simulink model "positionWalking_legacy"  (Simulink 8.3)
settings: Solver=FixedStepDiscrete  StartTime=0.0  StopTime=Config.t_end  FixedStep=Config.t_step  RelTol=1e-3
InitFcn:
  | cd(fileparts(which(bdroot)));
  | initTorqueWalking;
undefined symbols (not defined in the file): Config, DiscIntNeverNeededParam, gains, ROBOT_DOF
libraries: WBToolboxLibrary x88
(part 1 of 3)
settings Model: Creator=gnava  LastModifiedBy=gabri
settings DataIOCC: LimitDataPoints=off  SaveFormat=StructureWithTime  SignalLoggingSaveFormat=Dataset
settings DebuggingCC: UnderspecifiedInitializationDetection=Simplified  MergeDetectMultiDrivingBlocksExec=error  SolverPrmCheckMsg=none  FrameProcessingCompatibilityMsg=error  StateNameClashWarn=none  SFUnexpectedBacktrackingDiag=error  SFNoUnconditionalDefaultTransitionDiag=error
settings HardwareCC: ProdBitPerPointer=64  ProdLargestAtomicFloat=Float  ProdIntDivRoundTo=Zero  ProdEndianess=LittleEndian  ProdHWDeviceType=Specified
settings ModelReferenceCC: PropagateSignalLabelsOutOfModel=on
settings GRTTargetCC: TargetLangStandard=C99 (ISO)  GeneratePreprocessorConditionals=Use local settings  CombineOutputUpdateFcns=on  GRTInterface=off

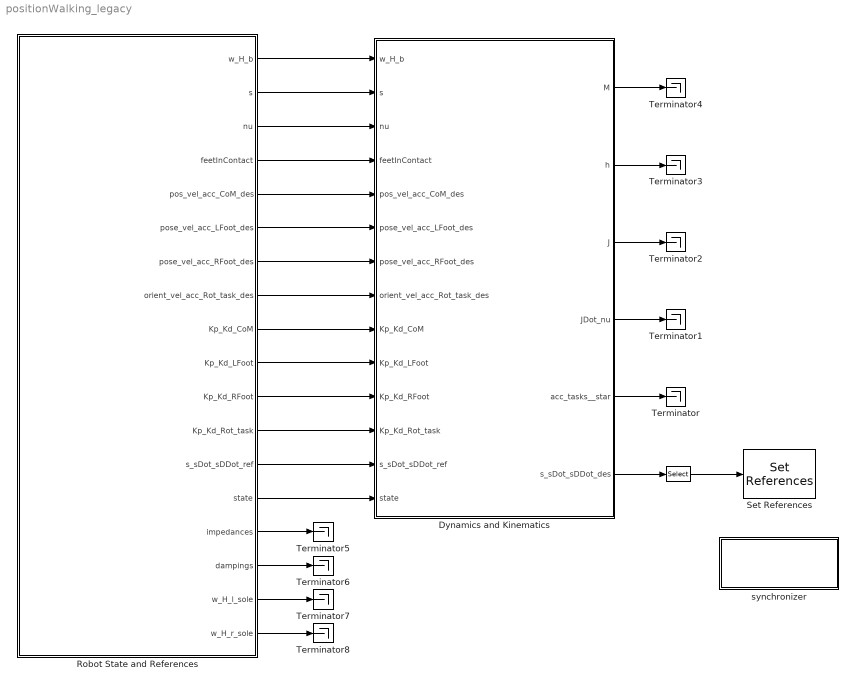
== system positionWalking_legacy ==
  "  " : Selector  NumberOfDimensions=2  InputPortWidth=ROBOT_DOF+16  IndexOptions=Index vector (dialog),Index vector (dialog)  Indices=[1:ROBOT_DOF],[1]  OutputSizes=1,1
  Dynamics and Kinematics : Subsystem
  Robot State and References : Subsystem
  Set References : WBToolboxLibrary/wholeBodyActuators/Set References  controlType=Position Direct  fullOrSubControl=Full  controlledJoints=''  robotName=WBT_robotName  localName=WBT_modelName  wbiFile=WBT_wbiFilename  wbiList=WBT_wbiList
  Terminator{,1..8} (9 alike) : Terminator
  synchronizer : Subsystem
      mask Display: disp('SYNCHRONIZER')
  wires:
  "  "/1 -> Set References/1
  Robot State and References/1(w_H_b) -> Dynamics and Kinematics/1(w_H_b)
  Robot State and References/2(s) -> Dynamics and Kinematics/2(s)
  Robot State and References/3(nu) -> Dynamics and Kinematics/3(nu)
  Robot State and References/4(feetInContact) -> Dynamics and Kinematics/4(feetInContact)
  Robot State and References/5(pos_vel_acc_CoM_des) -> Dynamics and Kinematics/5(pos_vel_acc_CoM_des)
  Robot State and References/6(pose_vel_acc_LFoot_des) -> Dynamics and Kinematics/6(pose_vel_acc_LFoot_des)
  Robot State and References/7(pose_vel_acc_RFoot_des) -> Dynamics and Kinematics/7(pose_vel_acc_RFoot_des)
  Robot State and References/8(orient_vel_acc_Rot_task_des) -> Dynamics and Kinematics/8(orient_vel_acc_Rot_task_des)
  Robot State and References/9(Kp_Kd_CoM) -> Dynamics and Kinematics/9(Kp_Kd_CoM)
  Robot State and References/10(Kp_Kd_LFoot) -> Dynamics and Kinematics/10(Kp_Kd_LFoot)
  Robot State and References/11(Kp_Kd_RFoot) -> Dynamics and Kinematics/11(Kp_Kd_RFoot)
  Robot State and References/12(Kp_Kd_Rot_task) -> Dynamics and Kinematics/12(Kp_Kd_Rot_task)
  Robot State and References/13(s_sDot_sDDot_ref) -> Dynamics and Kinematics/13(s_sDot_sDDot_ref)
  Robot State and References/14(state) -> Dynamics and Kinematics/14(state)
  Robot State and References/15(impedances) -> Terminator5/1
  Robot State and References/16(dampings) -> Terminator6/1
  Robot State and References/17(w_H_l_sole) -> Terminator7/1
  Robot State and References/18(w_H_r_sole) -> Terminator8/1
  Dynamics and Kinematics/6(s_sDot_sDDot_des) -> "  "/1
  Dynamics and Kinematics/5(acc_tasks__star) -> Terminator/1
  Dynamics and Kinematics/4(JDot_nu) -> Terminator1/1
  Dynamics and Kinematics/3(J) -> Terminator2/1
  Dynamics and Kinematics/2(h) -> Terminator3/1
  Dynamics and Kinematics/1(M) -> Terminator4/1

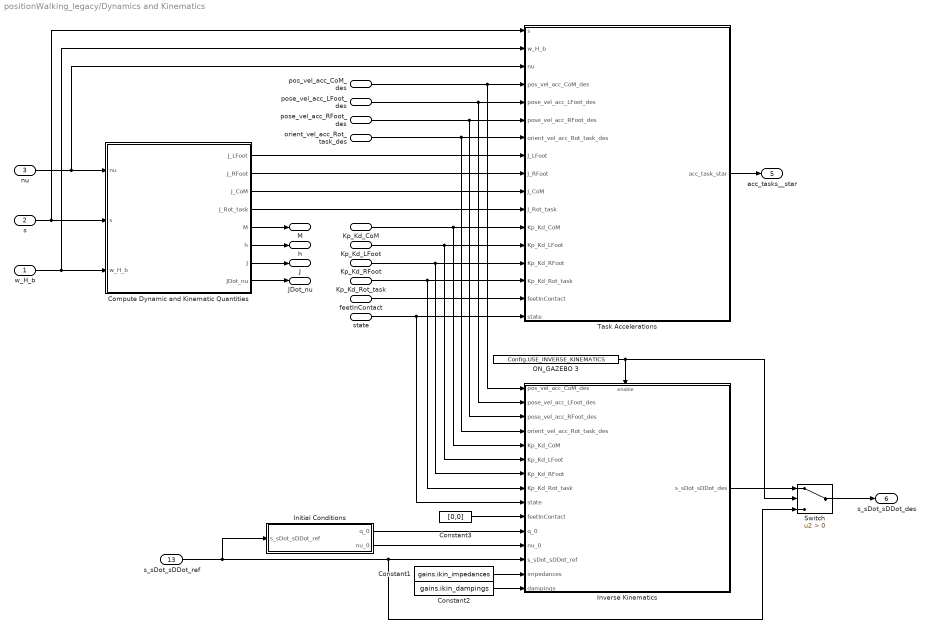
== system positionWalking_legacy/Dynamics and Kinematics ==
  w_H_b : Inport
  s : Inport  Port=2
  nu : Inport  Port=3
  feetInContact : Inport  Port=4
  pos_vel_acc_CoM_des : Inport  Port=5
  pose_vel_acc_LFoot_des : Inport  Port=6
  pose_vel_acc_RFoot_des : Inport  Port=7
  orient_vel_acc_Rot_task_des : Inport  Port=8
  Kp_Kd_CoM : Inport  Port=9
  Kp_Kd_LFoot : Inport  Port=10
  Kp_Kd_RFoot : Inport  Port=11
  Kp_Kd_Rot_task : Inport  Port=12
  s_sDot_sDDot_ref : Inport  Port=13
  state : Inport  Port=14
  Compute Dynamic and Kinematic Quantities : Subsystem
  Constant1 : Constant  Value=gains.ikin_impedances
  Constant2 : Constant  Value=gains.ikin_dampings
  Constant3 : Constant  Value=[0,0]
  Initial Conditions : Subsystem
  Inverse Kinematics : Subsystem
  ON_GAZEBO 3 : Constant  Value=Config.USE_INVERSE_KINEMATICS
  Switch : Switch  Criteria=u2 > Threshold
  Task Accelerations : Subsystem
  M : Outport
  h : Outport  Port=2
  J : Outport  Port=3
  JDot_nu : Outport  Port=4
  acc_tasks__star : Outport  Port=5
  s_sDot_sDDot_des : Outport  Port=6
  wires:
  pos_vel_acc_CoM_des/1 -> Inverse Kinematics/1(pos_vel_acc_CoM_des), Task Accelerations/4(pos_vel_acc_CoM_des)
  pose_vel_acc_LFoot_des/1 -> Inverse Kinematics/2(pose_vel_acc_LFoot_des), Task Accelerations/5(pose_vel_acc_LFoot_des)
  pose_vel_acc_RFoot_des/1 -> Inverse Kinematics/3(pose_vel_acc_RFoot_des), Task Accelerations/6(pose_vel_acc_RFoot_des)
  orient_vel_acc_Rot_task_des/1 -> Inverse Kinematics/4(orient_vel_acc_Rot_task_des), Task Accelerations/7(orient_vel_acc_Rot_task_des)
  Kp_Kd_CoM/1 -> Inverse Kinematics/5(Kp_Kd_CoM), Task Accelerations/12(Kp_Kd_CoM)
  Kp_Kd_LFoot/1 -> Inverse Kinematics/6(Kp_Kd_LFoot), Task Accelerations/13(Kp_Kd_LFoot)
  Kp_Kd_RFoot/1 -> Inverse Kinematics/7(Kp_Kd_RFoot), Task Accelerations/14(Kp_Kd_RFoot)
  Kp_Kd_Rot_task/1 -> Inverse Kinematics/8(Kp_Kd_Rot_task), Task Accelerations/15(Kp_Kd_Rot_task)
  feetInContact/1 -> Task Accelerations/16(feetInContact)
  Task Accelerations/1(acc_task_star) -> acc_tasks__star/1
  ON_GAZEBO 3/1 -> Switch/2, Inverse Kinematics/Enable
  Inverse Kinematics/1(s_sDot_sDDot_des) -> Switch/1
  state/1 -> Inverse Kinematics/9(state), Task Accelerations/17(state)
  nu/1 -> Compute Dynamic and Kinematic Quantities/1(nu), Task Accelerations/3(nu)
  s/1 -> Task Accelerations/1(s), Compute Dynamic and Kinematic Quantities/2(s)
  w_H_b/1 -> Compute Dynamic and Kinematic Quantities/3(w_H_b), Task Accelerations/2(w_H_b)
  Compute Dynamic and Kinematic Quantities/6(h) -> h/1
  Compute Dynamic and Kinematic Quantities/1(J_LFoot) -> Task Accelerations/8(J_LFoot)
  Compute Dynamic and Kinematic Quantities/2(J_RFoot) -> Task Accelerations/9(J_RFoot)
  Compute Dynamic and Kinematic Quantities/3(J_CoM) -> Task Accelerations/10(J_CoM)
  Compute Dynamic and Kinematic Quantities/5(M) -> M/1
  Compute Dynamic and Kinematic Quantities/4(J_Rot_task) -> Task Accelerations/11(J_Rot_task)
  Compute Dynamic and Kinematic Quantities/7(J) -> J/1
  Compute Dynamic and Kinematic Quantities/8(JDot_nu) -> JDot_nu/1
  s_sDot_sDDot_ref/1 -> Inverse Kinematics/13(s_sDot_sDDot_ref), Switch/3, Initial Conditions/1(s_sDot_sDDot_ref)
  Initial Conditions/1(q_0) -> Inverse Kinematics/11(q_0)
  Initial Conditions/2(nu_0) -> Inverse Kinematics/12(nu_0)
  Constant1/1 -> Inverse Kinematics/14(impedances)
  Constant2/1 -> Inverse Kinematics/15(dampings)
  Switch/1 -> s_sDot_sDDot_des/1
  Constant3/1 -> Inverse Kinematics/10(feetInContact)

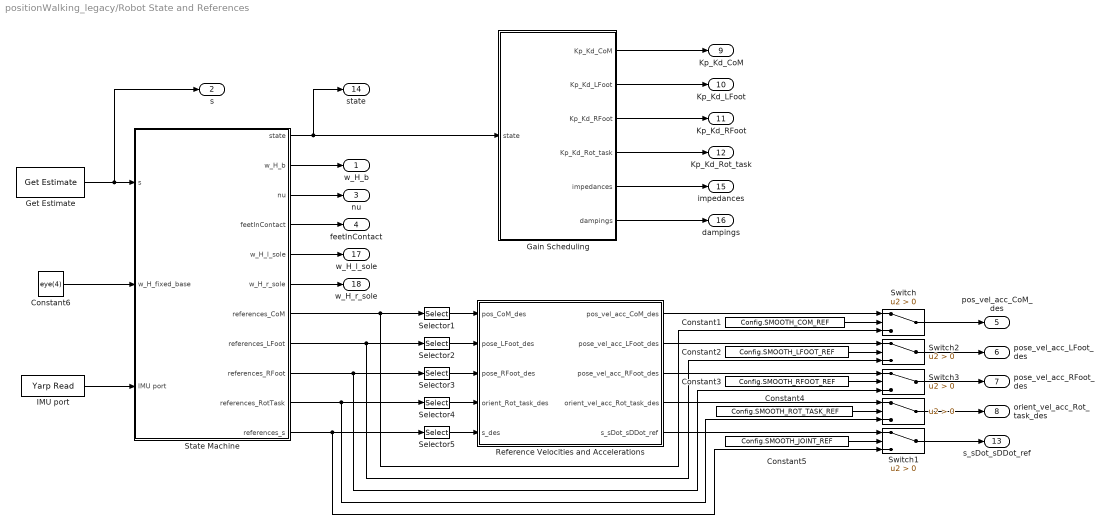
== system positionWalking_legacy/Robot State and References ==
  " " : Switch  Criteria=u2 > Threshold
  Constant1 : Constant  Value=Config.SMOOTH_COM_REF
  Constant2 : Constant  Value=Config.SMOOTH_LFOOT_REF
  Constant3 : Constant  Value=Config.SMOOTH_RFOOT_REF
  Constant4 : Constant  Value=Config.SMOOTH_ROT_TASK_REF
  Constant5 : Constant  Value=Config.SMOOTH_JOINT_REF
  Constant6 : Constant  Value=eye(4)
  Gain Scheduling : Subsystem
  Get Estimate : WBToolboxLibrary/wholeBodyStates/Get Estimate  estimateType=Joints Position  robotName=WBT_robotName  localName=WBT_modelName  wbiFile=WBT_wbiFilename  wbiList=WBT_wbiList
  IMU port : WBToolboxLibrary/Utilities/Yarp Read  portName=Ports.IMU  signalSize=12  blocking=off  timestamp=off  autoconnect=on  errorOnConnection=off
  Reference Velocities and Accelerations : Subsystem
  Selector1 : Selector  NumberOfDimensions=2  InputPortWidth=3  IndexOptions=Index vector (dialog),Index vector (dialog)  Indices=[1:3],1  OutputSizes=1,1
  Selector2 : Selector  NumberOfDimensions=2  InputPortWidth=3  IndexOptions=Index vector (dialog),Index vector (dialog)  Indices=[1:6],[1:3]  OutputSizes=1,1
  Selector3 : Selector  NumberOfDimensions=2  InputPortWidth=3  IndexOptions=Index vector (dialog),Index vector (dialog)  Indices=[1:6],[1:3]  OutputSizes=1,1
  Selector4 : Selector  NumberOfDimensions=2  InputPortWidth=3  IndexOptions=Index vector (dialog),Index vector (dialog)  Indices=[1:3],[1:3]  OutputSizes=1,1
  Selector5 : Selector  NumberOfDimensions=2  InputPortWidth=ROBOT_DOF  IndexOptions=Index vector (dialog),Index vector (dialog)  Indices=[1:ROBOT_DOF],1  OutputSizes=1,1
  State Machine : Subsystem
  Switch{,1..3} (4 alike) : Switch  Criteria=u2 > Threshold
  w_H_b : Outport
  s : Outport  Port=2
  nu : Outport  Port=3
  feetInContact : Outport  Port=4
  pos_vel_acc_CoM_des : Outport  Port=5
  pose_vel_acc_LFoot_des : Outport  Port=6
  pose_vel_acc_RFoot_des : Outport  Port=7
  orient_vel_acc_Rot_task_des : Outport  Port=8
  Kp_Kd_CoM : Outport  Port=9
  Kp_Kd_LFoot : Outport  Port=10
  Kp_Kd_RFoot : Outport  Port=11
  Kp_Kd_Rot_task : Outport  Port=12
  s_sDot_sDDot_ref : Outport  Port=13
  state : Outport  Port=14
  impedances : Outport  Port=15
  dampings : Outport  Port=16
  w_H_l_sole : Outport  Port=17
  w_H_r_sole : Outport  Port=18
  wires:
  Gain Scheduling/1(Kp_Kd_CoM) -> Kp_Kd_CoM/1
  Gain Scheduling/2(Kp_Kd_LFoot) -> Kp_Kd_LFoot/1
  Gain Scheduling/3(Kp_Kd_RFoot) -> Kp_Kd_RFoot/1
  Gain Scheduling/4(Kp_Kd_Rot_task) -> Kp_Kd_Rot_task/1
  Gain Scheduling/5(impedances) -> impedances/1
  Gain Scheduling/6(dampings) -> dampings/1
  State Machine/1(state) -> state/1, Gain Scheduling/1(state)
  State Machine/4(feetInContact) -> feetInContact/1
  State Machine/3(nu) -> nu/1
  Constant6/1 -> State Machine/2(w_H_fixed_base)
  Get Estimate/1 -> s/1, State Machine/1(s)
  IMU port/1 -> State Machine/3(IMU port)
  State Machine/7(references_CoM) -> Selector1/1, Switch/3
  State Machine/2(w_H_b) -> w_H_b/1
  State Machine/8(references_LFoot) -> Selector2/1, Switch2/3
  State Machine/9(references_RFoot) -> Selector3/1, Switch3/3
  State Machine/10(references_RotTask) -> Selector4/1, " "/3
  State Machine/11(references_s) -> Selector5/1, Switch1/3
  State Machine/5(w_H_l_sole) -> w_H_l_sole/1
  State Machine/6(w_H_r_sole) -> w_H_r_sole/1
  Selector1/1 -> Reference Velocities and Accelerations/1(pos_CoM_des)
  Selector2/1 -> Reference Velocities and Accelerations/2(pose_LFoot_des)
  Selector3/1 -> Reference Velocities and Accelerations/3(pose_RFoot_des)
  Selector4/1 -> Reference Velocities and Accelerations/4(orient_Rot_task_des)
  Selector5/1 -> Reference Velocities and Accelerations/5(s_des)
  Switch3/1 -> pose_vel_acc_RFoot_des/1
  Switch2/1 -> pose_vel_acc_LFoot_des/1
  Switch1/1 -> s_sDot_sDDot_ref/1
  " "/1 -> orient_vel_acc_Rot_task_des/1
  Reference Velocities and Accelerations/1(pos_vel_acc_CoM_des) -> Switch/1
  Reference Velocities and Accelerations/4(orient_vel_acc_Rot_task_des) -> " "/1
  Reference Velocities and Accelerations/5(s_sDot_sDDot_ref) -> Switch1/1
  Reference Velocities and Accelerations/2(pose_vel_acc_LFoot_des) -> Switch2/1
  Reference Velocities and Accelerations/3(pose_vel_acc_RFoot_des) -> Switch3/1
  Constant1/1 -> Switch/2
  Constant3/1 -> Switch3/2
  Constant2/1 -> Switch2/2
  Constant5/1 -> Switch1/2
  Constant4/1 -> " "/2
  Switch/1 -> pos_vel_acc_CoM_des/1

== system positionWalking_legacy/synchronizer ==
  GAZEBO_SYNCHRONIZER : Subsystem
  Logical Operator : Logic  Operator=NOT  AllPortsSameDT=off  OutDataTypeStr=boolean
  "ON_GAZEBO " : Constant  Value=Config.ON_GAZEBO
  REAL_TIME_SYNC : Subsystem
  wires:
  Logical Operator/1 -> REAL_TIME_SYNC/Enable
  "ON_GAZEBO "/1 -> Logical Operator/1, GAZEBO_SYNCHRONIZER/Enable

== system positionWalking_legacy/Dynamics and Kinematics/Compute Dynamic and Kinematic Quantities ==
  nu : Inport
  s : Inport  Port=2
  w_H_b : Inport  Port=3
  "  " : Selector  NumberOfDimensions=2  InputPortWidth=ROBOT_DOF+16  IndexOptions=Index vector (dialog),Index vector (dialog)  Indices=[1:3],[1:ROBOT_DOF+6]  OutputSizes=1,1
  "   " : Selector  InputPortWidth=6  IndexOptions=Index vector (dialog)  Indices=[1:3]  OutputSizes=1
  "     " : Selector  NumberOfDimensions=2  InputPortWidth=ROBOT_DOF+16  IndexOptions=Index vector (dialog),Index vector (dialog)  Indices=[4:6],[1:ROBOT_DOF+6]  OutputSizes=1,1
  "               " : Selector  InputPortWidth=6  IndexOptions=Index vector (dialog)  Indices=[4:6]  OutputSizes=1
  Jacobians and JDot_nu : Subsystem
  Mass Matrix and Bias Forces : Subsystem
  Matrix Concatenate : Concatenate  NumInputs=4  Mode=Multidimensional array
  Selector : Selector  InputPortWidth=ROBOT_DOF+6  IndexOptions=Index vector (dialog)  Indices=[1:6]  OutputSizes=1
  Selector1 : Selector  InputPortWidth=ROBOT_DOF+6  IndexOptions=Index vector (dialog)  Indices=[7:ROBOT_DOF+6]  OutputSizes=1
  Vector Concatenate : Concatenate  NumInputs=4
  J_LFoot : Outport
  J_RFoot : Outport  Port=2
  J_CoM : Outport  Port=3
  J_Rot_task : Outport  Port=4
  M : Outport  Port=5
  h : Outport  Port=6
  J : Outport  Port=7
  JDot_nu : Outport  Port=8
  wires:
  "               "/1 -> Vector Concatenate/4
  "  "/1 -> J_CoM/1, Matrix Concatenate/3
  "     "/1 -> J_Rot_task/1, Matrix Concatenate/4
  Vector Concatenate/1 -> JDot_nu/1
  Selector1/1 -> Mass Matrix and Bias Forces/3(sDot), Jacobians and JDot_nu/3(sDot)
  Matrix Concatenate/1 -> J/1
  nu/1 -> Selector/1, Selector1/1
  Selector/1 -> Mass Matrix and Bias Forces/2(nu_b), Jacobians and JDot_nu/2(nu_b)
  "   "/1 -> Vector Concatenate/3
  Mass Matrix and Bias Forces/2(M(q)) -> M/1
  Mass Matrix and Bias Forces/1(h(q,nu)) -> h/1
  s/1 -> Jacobians and JDot_nu/1(s), Mass Matrix and Bias Forces/1(s)
  w_H_b/1 -> Jacobians and JDot_nu/4(w_H_b), Mass Matrix and Bias Forces/4(w_H_b)
  Jacobians and JDot_nu/2(J_RFoot) -> J_RFoot/1, Matrix Concatenate/2
  Jacobians and JDot_nu/1(J_LFoot) -> J_LFoot/1, Matrix Concatenate/1
  Jacobians and JDot_nu/3(J_CoM) -> "  "/1
  Jacobians and JDot_nu/4(J_Rot_task) -> "     "/1
  Jacobians and JDot_nu/5(JDot_nu_LFoot) -> Vector Concatenate/1
  Jacobians and JDot_nu/6(JDot_nu_RFoot) -> Vector Concatenate/2
  Jacobians and JDot_nu/7(JDot_nu_CoM) -> "   "/1
  Jacobians and JDot_nu/8(JDot_nu_Rot_task) -> "               "/1

== system positionWalking_legacy/Dynamics and Kinematics/Initial Conditions ==
  s_sDot_sDDot_ref : Inport
  "   2" : WBToolboxLibrary/Utilities/holder 
  Constant1 : Constant  Value=[1;1]
  Constant6 : Constant  Value=eye(4)
  "Inv\\*  " : Product  Inputs=/*  Multiplication=Matrix(*)
  Mux : Mux  Inputs=2
  Reshape : Reshape
  Selector : Selector  NumberOfDimensions=2  InputPortWidth=3  IndexOptions=Index vector (dialog),Index vector (dialog)  Indices=[1:ROBOT_DOF],1  OutputSizes=1,1
  Selector1 : Selector  NumberOfDimensions=2  InputPortWidth=3  IndexOptions=Index vector (dialog),Index vector (dialog)  Indices=[1:ROBOT_DOF],2  OutputSizes=1,1
  compute state velocity : Subsystem
  left foot : WBToolboxLibrary/wholeBodyModel/Kinematics/Forward Kinematics  frameName=Frames.LEFT_FOOT  robotName=WBT_robotName  localName=WBT_modelName  wbiFile=WBT_wbiFilename  wbiList=WBT_wbiList
  root_link : WBToolboxLibrary/wholeBodyModel/Kinematics/Forward Kinematics  frameName='root_link'  robotName=WBT_robotName  localName=WBT_modelName  wbiFile=WBT_wbiFilename  wbiList=WBT_wbiList
  q_0 : Outport
  nu_0 : Outport  Port=2
  wires:
  Reshape/1 -> Mux/1
  Mux/1 -> q_0/1
  s_sDot_sDDot_ref/1 -> "   2"/1
  Constant6/1 -> left foot/1, root_link/1
  left foot/1 -> "Inv\\*  "/1
  root_link/1 -> "Inv\\*  "/2
  "Inv\\*  "/1 -> compute state velocity/2(w_H_b), Reshape/1
  "   2"/1 -> Selector/1, Selector1/1
  Selector/1 -> left foot/2, root_link/2, compute state velocity/1(s), Mux/2
  Constant1/1 -> compute state velocity/3("feetInContact ")
  compute state velocity/1(nu) -> nu_0/1
  Selector1/1 -> compute state velocity/4("sDot ")

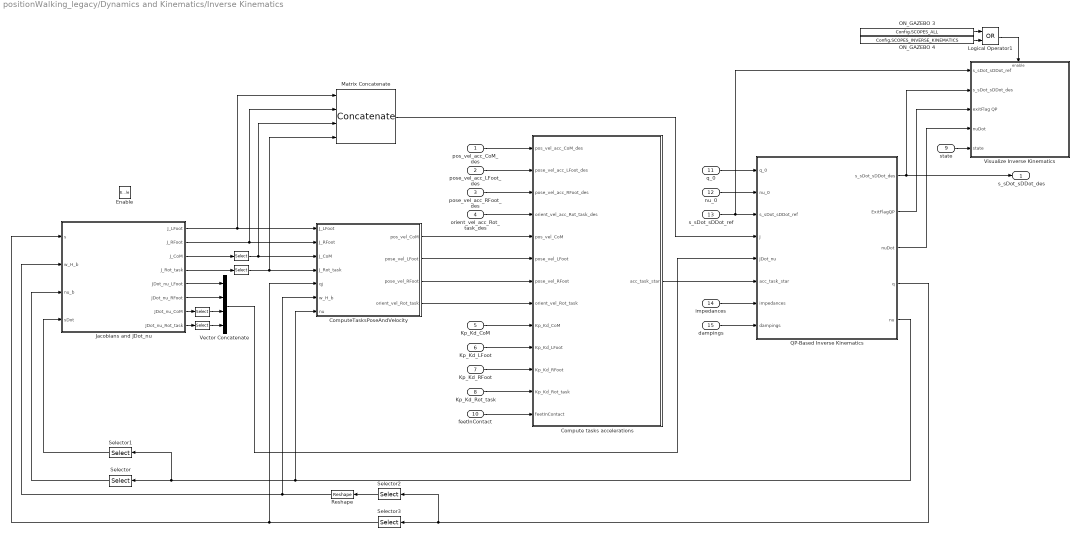
== system positionWalking_legacy/Dynamics and Kinematics/Inverse Kinematics ==
  pos_vel_acc_CoM_des : Inport
  pose_vel_acc_LFoot_des : Inport  Port=2
  pose_vel_acc_RFoot_des : Inport  Port=3
  orient_vel_acc_Rot_task_des : Inport  Port=4
  Kp_Kd_CoM : Inport  Port=5
  Kp_Kd_LFoot : Inport  Port=6
  Kp_Kd_RFoot : Inport  Port=7
  Kp_Kd_Rot_task : Inport  Port=8
  state : Inport  Port=9
  feetInContact : Inport  Port=10
  q_0 : Inport  Port=11
  nu_0 : Inport  Port=12
  s_sDot_sDDot_ref : Inport  Port=13
  impedances : Inport  Port=14
  dampings : Inport  Port=15
  Enable : EnablePort
  "  " : Selector  NumberOfDimensions=2  InputPortWidth=ROBOT_DOF+16  IndexOptions=Index vector (dialog),Index vector (dialog)  Indices=[1:3],[1:ROBOT_DOF+6]  OutputSizes=1,1
  "   " : Selector  InputPortWidth=6  IndexOptions=Index vector (dialog)  Indices=[1:3]  OutputSizes=1
  "     " : Selector  NumberOfDimensions=2  InputPortWidth=ROBOT_DOF+16  IndexOptions=Index vector (dialog),Index vector (dialog)  Indices=[4:6],[1:ROBOT_DOF+6]  OutputSizes=1,1
  "               " : Selector  InputPortWidth=6  IndexOptions=Index vector (dialog)  Indices=[4:6]  OutputSizes=1
  Compute tasks accelerations : MATLAB Function  TreatAsAtomicUnit=on
      settings: PermitHierarchicalResolution=ParametersOnly
  ComputeTasksPoseAndVelocity : Subsystem
  Jacobians and JDot_nu : Subsystem
  Logical Operator1 : Logic  Operator=OR  AllPortsSameDT=off  OutDataTypeStr=boolean
  Matrix Concatenate : Concatenate  NumInputs=4  Mode=Multidimensional array
  ON_GAZEBO 3 : Constant  Value=Config.SCOPES_ALL
  ON_GAZEBO 4 : Constant  Value=Config.SCOPES_INVERSE_KINEMATICS
  QP-Based Inverse Kinematics : Subsystem
  Reshape : Reshape  OutputDimensionality=Customize  OutputDimensions=[4,4]
  Selector : Selector  InputPortWidth=ROBOT_DOF+6  IndexOptions=Index vector (dialog)  Indices=[1:6]  OutputSizes=1
  Selector1 : Selector  InputPortWidth=ROBOT_DOF+6  IndexOptions=Index vector (dialog)  Indices=[7:ROBOT_DOF+6]  OutputSizes=1
  Selector2 : Selector  InputPortWidth=ROBOT_DOF+16  IndexOptions=Index vector (dialog)  Indices=[1:16]  OutputSizes=1
  Selector3 : Selector  InputPortWidth=ROBOT_DOF+16  IndexOptions=Index vector (dialog)  Indices=[17:ROBOT_DOF+16]  OutputSizes=1
  Vector Concatenate : Concatenate  NumInputs=4
  Visualize Inverse Kinematics : Subsystem
  s_sDot_sDDot_des : Outport
  wires:
  Kp_Kd_CoM/1 -> Compute tasks accelerations/9(Kp_Kd_CoM)
  Kp_Kd_LFoot/1 -> Compute tasks accelerations/10(Kp_Kd_LFoot)
  pose_vel_acc_LFoot_des/1 -> Compute tasks accelerations/2(pose_vel_acc_LFoot_des)
  Kp_Kd_RFoot/1 -> Compute tasks accelerations/11(Kp_Kd_RFoot)
  orient_vel_acc_Rot_task_des/1 -> Compute tasks accelerations/4(orient_vel_acc_Rot_task_des)
  pose_vel_acc_RFoot_des/1 -> Compute tasks accelerations/3(pose_vel_acc_RFoot_des)
  Kp_Kd_Rot_task/1 -> Compute tasks accelerations/12(Kp_Kd_Rot_task)
  pos_vel_acc_CoM_des/1 -> Compute tasks accelerations/1(pos_vel_acc_CoM_des)
  ComputeTasksPoseAndVelocity/1(pos_vel_CoM) -> Compute tasks accelerations/5(pos_vel_CoM)
  ComputeTasksPoseAndVelocity/2(pose_vel_LFoot) -> Compute tasks accelerations/6(pose_vel_LFoot)
  ComputeTasksPoseAndVelocity/3(pose_vel_RFoot) -> Compute tasks accelerations/7(pose_vel_RFoot)
  ComputeTasksPoseAndVelocity/4(orient_vel_Rot_task) -> Compute tasks accelerations/8(orient_vel_Rot_task)
  s_sDot_sDDot_ref/1 -> Visualize Inverse Kinematics/1(s_sDot_sDDot_ref), QP-Based Inverse Kinematics/3(s_sDot_sDDot_ref)
  Selector2/1 -> Reshape/1
  "  "/1 -> ComputeTasksPoseAndVelocity/3(J_CoM), Matrix Concatenate/3
  "   "/1 -> Vector Concatenate/3
  ON_GAZEBO 4/1 -> Logical Operator1/2
  ON_GAZEBO 3/1 -> Logical Operator1/1
  Jacobians and JDot_nu/2(J_RFoot) -> Matrix Concatenate/2, ComputeTasksPoseAndVelocity/2(J_RFoot)
  Jacobians and JDot_nu/1(J_LFoot) -> Matrix Concatenate/1, ComputeTasksPoseAndVelocity/1(J_LFoot)
  Selector1/1 -> Jacobians and JDot_nu/4(sDot)
  Selector/1 -> Jacobians and JDot_nu/3(nu_b)
  Jacobians and JDot_nu/4(J_Rot_task) -> "     "/1
  Jacobians and JDot_nu/5(JDot_nu_LFoot) -> Vector Concatenate/1
  Jacobians and JDot_nu/6(JDot_nu_RFoot) -> Vector Concatenate/2
  Jacobians and JDot_nu/7(JDot_nu_CoM) -> "   "/1
  Jacobians and JDot_nu/8(JDot_nu_Rot_task) -> "               "/1
  Vector Concatenate/1 -> QP-Based Inverse Kinematics/5(JDot_nu)
  dampings/1 -> QP-Based Inverse Kinematics/8(dampings)
  Compute tasks accelerations/1(acc_task_star) -> QP-Based Inverse Kinematics/6(acc_task_star)
  impedances/1 -> QP-Based Inverse Kinematics/7(impedances)
  Matrix Concatenate/1 -> QP-Based Inverse Kinematics/4(J)
  nu_0/1 -> QP-Based Inverse Kinematics/2(nu_0)
  q_0/1 -> QP-Based Inverse Kinematics/1(q_0)
  QP-Based Inverse Kinematics/5(nu) -> ComputeTasksPoseAndVelocity/7(nu), Selector1/1, Selector/1
  QP-Based Inverse Kinematics/4(q) -> Selector2/1, Selector3/1
  state/1 -> Visualize Inverse Kinematics/5(state)
  QP-Based Inverse Kinematics/2(ExitFlagQP) -> Visualize Inverse Kinematics/3(exitFlag QP)
  QP-Based Inverse Kinematics/3(nuDot) -> Visualize Inverse Kinematics/4(nuDot)
  Logical Operator1/1 -> Visualize Inverse Kinematics/Enable
  QP-Based Inverse Kinematics/1(s_sDot_sDDot_des) -> s_sDot_sDDot_des/1, Visualize Inverse Kinematics/2(s_sDot_sDDot_des)
  "     "/1 -> Matrix Concatenate/4, ComputeTasksPoseAndVelocity/4(J_Rot_task)
  "               "/1 -> Vector Concatenate/4
  Jacobians and JDot_nu/3(J_CoM) -> "  "/1
  Reshape/1 -> Jacobians and JDot_nu/2(w_H_b), ComputeTasksPoseAndVelocity/6(w_H_b)
  Selector3/1 -> Jacobians and JDot_nu/1(s), ComputeTasksPoseAndVelocity/5(qj)
  feetInContact/1 -> Compute tasks accelerations/13(feetInContact)

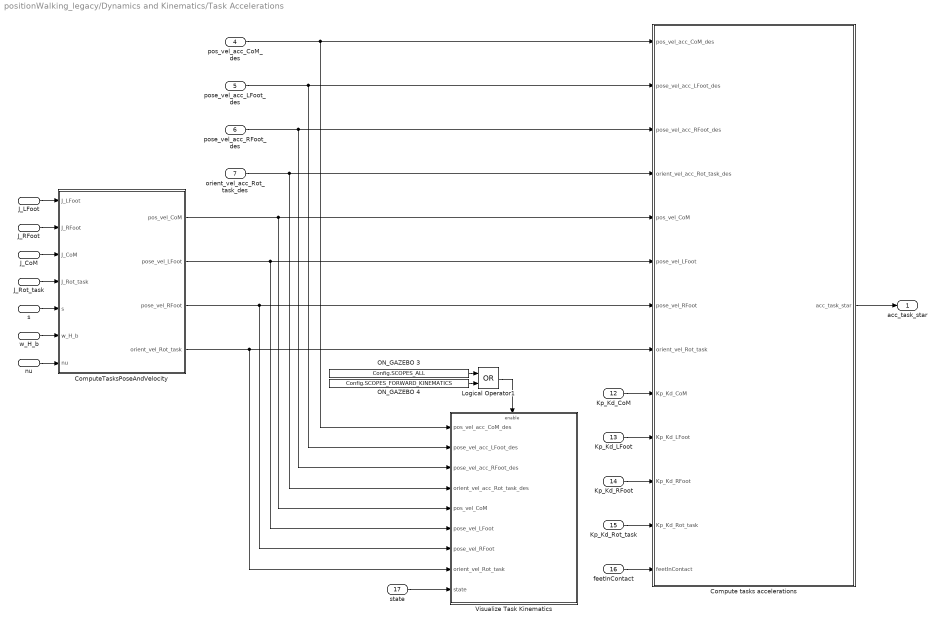
== system positionWalking_legacy/Dynamics and Kinematics/Task Accelerations ==
  s : Inport
  w_H_b : Inport  Port=2
  nu : Inport  Port=3
  pos_vel_acc_CoM_des : Inport  Port=4
  pose_vel_acc_LFoot_des : Inport  Port=5
  pose_vel_acc_RFoot_des : Inport  Port=6
  orient_vel_acc_Rot_task_des : Inport  Port=7
  J_LFoot : Inport  Port=8
  J_RFoot : Inport  Port=9
  J_CoM : Inport  Port=10
  J_Rot_task : Inport  Port=11
  Kp_Kd_CoM : Inport  Port=12
  Kp_Kd_LFoot : Inport  Port=13
  Kp_Kd_RFoot : Inport  Port=14
  Kp_Kd_Rot_task : Inport  Port=15
  feetInContact : Inport  Port=16
  state : Inport  Port=17
  Compute tasks accelerations : MATLAB Function  TreatAsAtomicUnit=on
      settings: PermitHierarchicalResolution=ParametersOnly
  ComputeTasksPoseAndVelocity : Subsystem
  Logical Operator1 : Logic  Operator=OR  AllPortsSameDT=off  OutDataTypeStr=boolean
  ON_GAZEBO 3 : Constant  Value=Config.SCOPES_ALL
  ON_GAZEBO 4 : Constant  Value=Config.SCOPES_FORWARD_KINEMATICS
  Visualize Task Kinematics : Subsystem
  acc_task_star : Outport
  wires:
  pos_vel_acc_CoM_des/1 -> Visualize Task Kinematics/1(pos_vel_acc_CoM_des), Compute tasks accelerations/1(pos_vel_acc_CoM_des)
  Kp_Kd_RFoot/1 -> Compute tasks accelerations/11(Kp_Kd_RFoot)
  Kp_Kd_Rot_task/1 -> Compute tasks accelerations/12(Kp_Kd_Rot_task)
  feetInContact/1 -> Compute tasks accelerations/13(feetInContact)
  pose_vel_acc_RFoot_des/1 -> Visualize Task Kinematics/3(pose_vel_acc_RFoot_des), Compute tasks accelerations/3(pose_vel_acc_RFoot_des)
  Kp_Kd_LFoot/1 -> Compute tasks accelerations/10(Kp_Kd_LFoot)
  Kp_Kd_CoM/1 -> Compute tasks accelerations/9(Kp_Kd_CoM)
  orient_vel_acc_Rot_task_des/1 -> Visualize Task Kinematics/4(orient_vel_acc_Rot_task_des), Compute tasks accelerations/4(orient_vel_acc_Rot_task_des)
  pose_vel_acc_LFoot_des/1 -> Visualize Task Kinematics/2(pose_vel_acc_LFoot_des), Compute tasks accelerations/2(pose_vel_acc_LFoot_des)
  Compute tasks accelerations/1(acc_task_star) -> acc_task_star/1
  ComputeTasksPoseAndVelocity/1(pos_vel_CoM) -> Visualize Task Kinematics/5(pos_vel_CoM), Compute tasks accelerations/5(pos_vel_CoM)
  ComputeTasksPoseAndVelocity/2(pose_vel_LFoot) -> Visualize Task Kinematics/6(pose_vel_LFoot), Compute tasks accelerations/6(pose_vel_LFoot)
  ComputeTasksPoseAndVelocity/3(pose_vel_RFoot) -> Visualize Task Kinematics/7(pose_vel_RFoot), Compute tasks accelerations/7(pose_vel_RFoot)
  ComputeTasksPoseAndVelocity/4(orient_vel_Rot_task) -> Visualize Task Kinematics/8(orient_vel_Rot_task), Compute tasks accelerations/8(orient_vel_Rot_task)
  J_LFoot/1 -> ComputeTasksPoseAndVelocity/1(J_LFoot)
  J_RFoot/1 -> ComputeTasksPoseAndVelocity/2(J_RFoot)
  J_CoM/1 -> ComputeTasksPoseAndVelocity/3(J_CoM)
  J_Rot_task/1 -> ComputeTasksPoseAndVelocity/4(J_Rot_task)
  s/1 -> ComputeTasksPoseAndVelocity/5(s)
  w_H_b/1 -> ComputeTasksPoseAndVelocity/6(w_H_b)
  nu/1 -> ComputeTasksPoseAndVelocity/7(nu)
  ON_GAZEBO 4/1 -> Logical Operator1/2
  ON_GAZEBO 3/1 -> Logical Operator1/1
  Logical Operator1/1 -> Visualize Task Kinematics/Enable
  state/1 -> Visualize Task Kinematics/9(state)

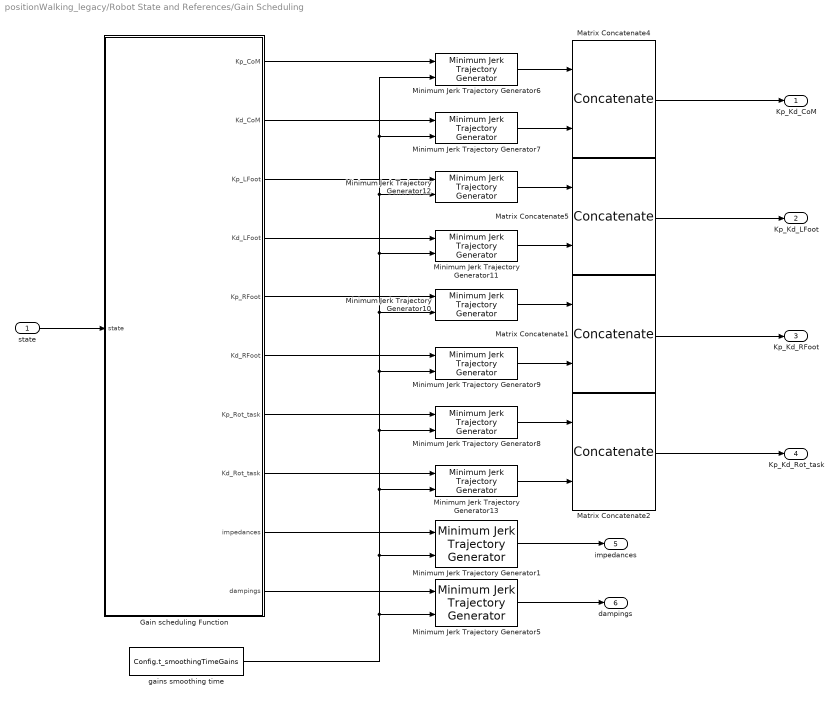
== system positionWalking_legacy/Robot State and References/Gain Scheduling ==
  state : Inport
  Gain scheduling Function : MATLAB Function  TreatAsAtomicUnit=on
      settings: PermitHierarchicalResolution=ParametersOnly
  Matrix Concatenate{1..2,4..5} (4 alike) : Concatenate  Mode=Multidimensional array  ConcatenateDimension=2
  Minimum Jerk Trajectory Generator{1,5..13} (10 alike) : WBToolboxLibrary/Utilities/Minimum Jerk Trajectory Generator  externalSettlingTime=on  settlingTime=3  sampleTime=Config.t_step  resetOnSettlingTime=off  firstDerivatives=off  secondDerivatives=off  explicitInitialValue=off
  gains smoothing time : Constant  Value=Config.t_smoothingTimeGains
  Kp_Kd_CoM : Outport
  Kp_Kd_LFoot : Outport  Port=2
  Kp_Kd_RFoot : Outport  Port=3
  Kp_Kd_Rot_task : Outport  Port=4
  impedances : Outport  Port=5
  dampings : Outport  Port=6
  wires:
  Matrix Concatenate5/1 -> Kp_Kd_LFoot/1
  Matrix Concatenate1/1 -> Kp_Kd_RFoot/1
  Matrix Concatenate2/1 -> Kp_Kd_Rot_task/1
  Matrix Concatenate4/1 -> Kp_Kd_CoM/1
  Minimum Jerk Trajectory Generator5/1 -> dampings/1
  Minimum Jerk Trajectory Generator1/1 -> impedances/1
  Gain scheduling Function/9(impedances) -> Minimum Jerk Trajectory Generator1/1
  Gain scheduling Function/10(dampings) -> Minimum Jerk Trajectory Generator5/1
  state/1 -> Gain scheduling Function/1(state)
  Minimum Jerk Trajectory Generator13/1 -> Matrix Concatenate2/2
  Minimum Jerk Trajectory Generator8/1 -> Matrix Concatenate2/1
  Minimum Jerk Trajectory Generator9/1 -> Matrix Concatenate1/2
  Minimum Jerk Trajectory Generator10/1 -> Matrix Concatenate1/1
  Minimum Jerk Trajectory Generator11/1 -> Matrix Concatenate5/2
  Minimum Jerk Trajectory Generator12/1 -> Matrix Concatenate5/1
  Minimum Jerk Trajectory Generator7/1 -> Matrix Concatenate4/2
  Minimum Jerk Trajectory Generator6/1 -> Matrix Concatenate4/1
  Gain scheduling Function/1(Kp_CoM) -> Minimum Jerk Trajectory Generator6/1
  Gain scheduling Function/2(Kd_CoM) -> Minimum Jerk Trajectory Generator7/1
  Gain scheduling Function/3(Kp_LFoot) -> Minimum Jerk Trajectory Generator12/1
  Gain scheduling Function/4(Kd_LFoot) -> Minimum Jerk Trajectory Generator11/1
  Gain scheduling Function/5(Kp_RFoot) -> Minimum Jerk Trajectory Generator10/1
  Gain scheduling Function/6(Kd_RFoot) -> Minimum Jerk Trajectory Generator9/1
  Gain scheduling Function/7(Kp_Rot_task) -> Minimum Jerk Trajectory Generator8/1
  Gain scheduling Function/8(Kd_Rot_task) -> Minimum Jerk Trajectory Generator13/1
  gains smoothing time/1 -> Minimum Jerk Trajectory Generator1/2, Minimum Jerk Trajectory Generator13/2, Minimum Jerk Trajectory Generator8/2, Minimum Jerk Trajectory Generator9/2, Minimum Jerk Trajectory Generator10/2, Minimum Jerk Trajectory Generator11/2, Minimum Jerk Trajectory Generator12/2, Minimum Jerk Trajectory Generator7/2, Minimum Jerk Trajectory Generator6/2, Minimum Jerk Trajectory Generator5/2

== system positionWalking_legacy/Robot State and References/Reference Velocities and Accelerations ==
  pos_CoM_des : Inport
  pose_LFoot_des : Inport  Port=2
  pose_RFoot_des : Inport  Port=3
  orient_Rot_task_des : Inport  Port=4
  s_des : Inport  Port=5
  Matrix Concatenate8 : Concatenate  Mode=Multidimensional array
  Matrix Concatenate9 : Concatenate  Mode=Multidimensional array
  Reference Orientations : Subsystem
  Reference Positions : Subsystem
  Selector : Selector  NumberOfDimensions=2  InputPortWidth=3  IndexOptions=Index vector (dialog),Index vector (dialog)  Indices=[1:3],1  OutputSizes=1,1
  Selector1 : Selector  NumberOfDimensions=2  InputPortWidth=3  IndexOptions=Index vector (dialog),Index vector (dialog)  Indices=[1:3],1  OutputSizes=1,1
  Selector2 : Selector  NumberOfDimensions=2  InputPortWidth=3  IndexOptions=Index vector (dialog),Index vector (dialog)  Indices=[4:6],[1:3]  OutputSizes=1,1
  Selector3 : Selector  NumberOfDimensions=2  InputPortWidth=3  IndexOptions=Index vector (dialog),Index vector (dialog)  Indices=[4:6],[1:3]  OutputSizes=1,1
  pos_vel_acc_CoM_des : Outport
  pose_vel_acc_LFoot_des : Outport  Port=2
  pose_vel_acc_RFoot_des : Outport  Port=3
  orient_vel_acc_Rot_task_des : Outport  Port=4
  s_sDot_sDDot_ref : Outport  Port=5
  wires:
  pos_CoM_des/1 -> Reference Positions/1(pos_CoM_des)
  pose_LFoot_des/1 -> Selector2/1, Selector1/1
  pose_RFoot_des/1 -> Selector3/1, Selector/1
  s_des/1 -> Reference Positions/4(s_des)
  Reference Positions/1(pos_vel_acc_CoM_des) -> pos_vel_acc_CoM_des/1
  Reference Positions/2(s_sDot_sDDot_ref) -> s_sDot_sDDot_ref/1
  Selector/1 -> Reference Positions/3(pos_RFoot_des)
  Selector1/1 -> Reference Positions/2(pos_LFoot_des)
  orient_Rot_task_des/1 -> Reference Orientations/3(w_R_Rot_task_des)
  Reference Orientations/3(orient_vel_acc_Rot_task_des) -> orient_vel_acc_Rot_task_des/1
  Reference Orientations/1(orient_vel_acc_LFoot_des) -> Matrix Concatenate9/2
  Matrix Concatenate8/1 -> pose_vel_acc_RFoot_des/1
  Reference Orientations/2(orient_vel_acc_RFoot_des) -> Matrix Concatenate8/2
  Matrix Concatenate9/1 -> pose_vel_acc_LFoot_des/1
  Selector3/1 -> Reference Orientations/2(w_R_RFoot_des)
  Selector2/1 -> Reference Orientations/1(w_R_LFoot_des)
  Reference Positions/4(pos_vel_acc_RFoot_des) -> Matrix Concatenate8/1
  Reference Positions/3(pos_vel_acc_LFoot_des) -> Matrix Concatenate9/1

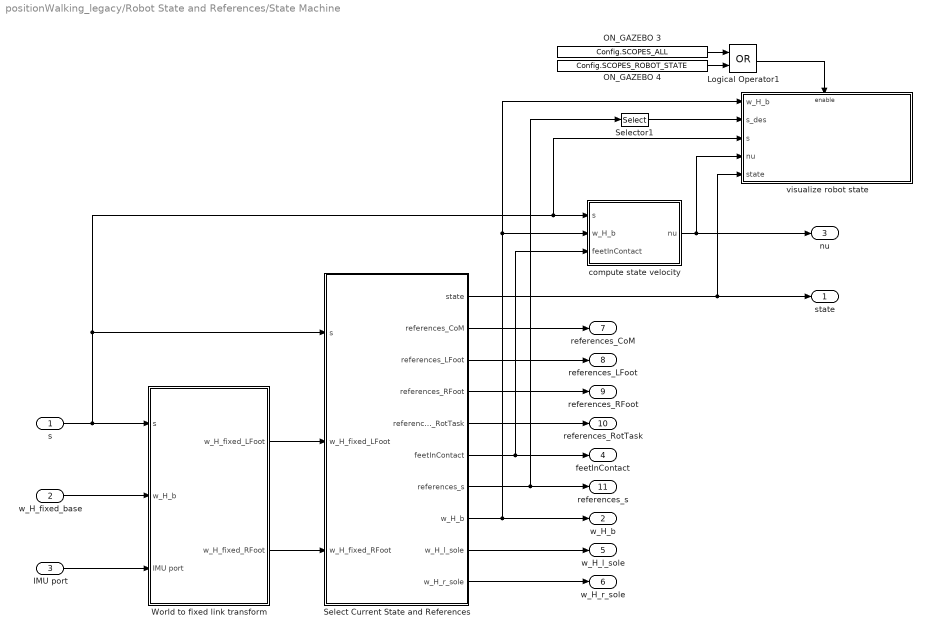
== system positionWalking_legacy/Robot State and References/State Machine ==
  s : Inport
  w_H_fixed_base : Inport  Port=2
  IMU port : Inport  Port=3
  Logical Operator1 : Logic  Operator=OR  AllPortsSameDT=off  OutDataTypeStr=boolean
  ON_GAZEBO 3 : Constant  Value=Config.SCOPES_ALL
  ON_GAZEBO 4 : Constant  Value=Config.SCOPES_ROBOT_STATE
  Select Current State and References : Subsystem
  Selector1 : Selector  NumberOfDimensions=2  InputPortWidth=ROBOT_DOF  IndexOptions=Index vector (dialog),Index vector (dialog)  Indices=[1:ROBOT_DOF],1  OutputSizes=1,1
  World to fixed link transform : Subsystem
  compute state velocity : Subsystem
  visualize robot state : Subsystem
  state : Outport
  w_H_b : Outport  Port=2
  nu : Outport  Port=3
  feetInContact : Outport  Port=4
  w_H_l_sole : Outport  Port=5
  w_H_r_sole : Outport  Port=6
  references_CoM : Outport  Port=7
  references_LFoot : Outport  Port=8
  references_RFoot : Outport  Port=9
  references_RotTask : Outport  Port=10
  references_s : Outport  Port=11
  wires:
  w_H_fixed_base/1 -> World to fixed link transform/2(w_H_b)
  s/1 -> compute state velocity/1(s), visualize robot state/3(s), Select Current State and References/1(s), World to fixed link transform/1(s)
  IMU port/1 -> World to fixed link transform/3(IMU port)
  compute state velocity/1(nu) -> nu/1, visualize robot state/4(nu)
  World to fixed link transform/1(w_H_fixed_LFoot) -> Select Current State and References/2(w_H_fixed_LFoot)
  World to fixed link transform/2(w_H_fixed_RFoot) -> Select Current State and References/3(w_H_fixed_RFoot)
  Select Current State and References/1(state) -> state/1, visualize robot state/5(state)
  Select Current State and References/2(references_CoM) -> references_CoM/1
  Select Current State and References/3(references_LFoot) -> references_LFoot/1
  Select Current State and References/4(references_RFoot) -> references_RFoot/1
  Select Current State and References/5(references_RotTask) -> references_RotTask/1
  Select Current State and References/6(feetInContact) -> feetInContact/1, compute state velocity/3("feetInContact ")
  Select Current State and References/8(w_H_b) -> visualize robot state/1(w_H_b), compute state velocity/2(w_H_b), w_H_b/1
  Select Current State and References/9(w_H_l_sole) -> w_H_l_sole/1
  Select Current State and References/10(w_H_r_sole) -> w_H_r_sole/1
  Select Current State and References/7(references_s) -> references_s/1, Selector1/1
  ON_GAZEBO 4/1 -> Logical Operator1/2
  ON_GAZEBO 3/1 -> Logical Operator1/1
  Logical Operator1/1 -> visualize robot state/Enable
  Selector1/1 -> visualize robot state/2(s_des)

== system positionWalking_legacy/synchronizer/GAZEBO_SYNCHRONIZER ==
  Enable : EnablePort
  Simulator Synchronizer : WBToolboxLibrary/Utilities/Simulator Synchronizer  period=Config.t_step  serverPortName='/clock/rpc'  clientPortName='/WBT_synchronizer/rpc:o'

== system positionWalking_legacy/synchronizer/REAL_TIME_SYNC ==
  Enable : EnablePort
  Real Time Synchronizer : WBToolboxLibrary/Utilities/Real Time Synchronizer  period=Config.t_step

== system positionWalking_legacy/Dynamics and Kinematics/Compute Dynamic and Kinematic Quantities/Jacobians and JDot_nu ==
  s : Inport
  nu_b : Inport  Port=2
  sDot : Inport  Port=3
  w_H_b : Inport  Port=4
  DotJ Nu : WBToolboxLibrary/wholeBodyModel/Jacobians/DotJ Nu  frameName=Frames.COM  robotName=WBT_robotName  localName=WBT_modelName  wbiFile=WBT_wbiFilename  wbiList=WBT_wbiList
  DotJ Nu1 : WBToolboxLibrary/wholeBodyModel/Jacobians/DotJ Nu  frameName=Frames.RIGHT_FOOT  robotName=WBT_robotName  localName=WBT_modelName  wbiFile=WBT_wbiFilename  wbiList=WBT_wbiList
  DotJ Nu2 : WBToolboxLibrary/wholeBodyModel/Jacobians/DotJ Nu  frameName=Frames.ROT_TASK_LINK  robotName=WBT_robotName  localName=WBT_modelName  wbiFile=WBT_wbiFilename  wbiList=WBT_wbiList
  DotJ Nu3 : WBToolboxLibrary/wholeBodyModel/Jacobians/DotJ Nu  frameName=Frames.LEFT_FOOT  robotName=WBT_robotName  localName=WBT_modelName  wbiFile=WBT_wbiFilename  wbiList=WBT_wbiList
  Jacobian CoM : WBToolboxLibrary/wholeBodyModel/Jacobians/Jacobian  frameName=Frames.COM  robotName=WBT_robotName  localName=WBT_modelName  wbiFile=WBT_wbiFilename  wbiList=WBT_wbiList
  Jacobian LFoot : WBToolboxLibrary/wholeBodyModel/Jacobians/Jacobian  frameName=Frames.LEFT_FOOT  robotName=WBT_robotName  localName=WBT_modelName  wbiFile=WBT_wbiFilename  wbiList=WBT_wbiList
  Jacobian RFoot : WBToolboxLibrary/wholeBodyModel/Jacobians/Jacobian  frameName=Frames.RIGHT_FOOT  robotName=WBT_robotName  localName=WBT_modelName  wbiFile=WBT_wbiFilename  wbiList=WBT_wbiList
  Jacobian Root Link : WBToolboxLibrary/wholeBodyModel/Jacobians/Jacobian  frameName=Frames.ROT_TASK_LINK  robotName=WBT_robotName  localName=WBT_modelName  wbiFile=WBT_wbiFilename  wbiList=WBT_wbiList
  J_LFoot : Outport
  J_RFoot : Outport  Port=2
  J_CoM : Outport  Port=3
  J_Rot_task : Outport  Port=4
  JDot_nu_LFoot : Outport  Port=5
  JDot_nu_RFoot : Outport  Port=6
  JDot_nu_CoM : Outport  Port=7
  JDot_nu_Rot_task : Outport  Port=8
  wires:
  Jacobian CoM/1 -> J_CoM/1
  Jacobian Root Link/1 -> J_Rot_task/1
  Jacobian LFoot/1 -> J_LFoot/1
  Jacobian RFoot/1 -> J_RFoot/1
  w_H_b/1 -> Jacobian RFoot/1, Jacobian LFoot/1, DotJ Nu1/1, DotJ Nu3/1, DotJ Nu2/1, DotJ Nu/1, Jacobian CoM/1, Jacobian Root Link/1
  sDot/1 -> DotJ Nu1/4, DotJ Nu3/4, DotJ Nu2/4, DotJ Nu/4
  nu_b/1 -> DotJ Nu/3, DotJ Nu1/3, DotJ Nu3/3, DotJ Nu2/3
  s/1 -> DotJ Nu1/2, DotJ Nu3/2, DotJ Nu2/2, DotJ Nu/2, Jacobian RFoot/2, Jacobian CoM/2, Jacobian Root Link/2, Jacobian LFoot/2
  DotJ Nu1/1 -> JDot_nu_RFoot/1
  DotJ Nu3/1 -> JDot_nu_LFoot/1
  DotJ Nu2/1 -> JDot_nu_Rot_task/1
  DotJ Nu/1 -> JDot_nu_CoM/1

== system positionWalking_legacy/Dynamics and Kinematics/Compute Dynamic and Kinematic Quantities/Mass Matrix and Bias Forces ==
  s : Inport
  nu_b : Inport  Port=2
  sDot : Inport  Port=3
  w_H_b : Inport  Port=4
  Get Bias Forces : WBToolboxLibrary/wholeBodyModel/Dynamics/Get Bias Forces  robotName=WBT_robotName  localName=WBT_modelName  wbiFile=WBT_wbiFilename  wbiList=WBT_wbiList  explicitGravity=off
  Mass Matrix : WBToolboxLibrary/wholeBodyModel/Dynamics/Mass Matrix  robotName=WBT_robotName  localName=WBT_modelName  wbiFile=WBT_wbiFilename  wbiList=WBT_wbiList
  h(q,nu) : Outport
  M(q) : Outport  Port=2
  wires:
  w_H_b/1 -> Mass Matrix/1, Get Bias Forces/1
  s/1 -> Mass Matrix/2, Get Bias Forces/2
  sDot/1 -> Get Bias Forces/4
  nu_b/1 -> Get Bias Forces/3
  Get Bias Forces/1 -> h(q,nu)/1
  Mass Matrix/1 -> M(q)/1

== system positionWalking_legacy/Dynamics and Kinematics/Initial Conditions/compute state velocity ==
  s : Inport
  w_H_b : Inport  Port=2
  "feetInContact " : Inport  Port=3
  "sDot " : Inport  Port=4
  Compute Base Velocity : MATLAB Function  TreatAsAtomicUnit=on
      settings: PermitHierarchicalResolution=ParametersOnly
  Feet Jacobians : Subsystem
  Mux : Mux  Inputs=2
  nu : Outport
  wires:
  "sDot "/1 -> Mux/2, Compute Base Velocity/4(sDot)
  Mux/1 -> nu/1
  "feetInContact "/1 -> Compute Base Velocity/3(feetInContact)
  Compute Base Velocity/1(nu_b) -> Mux/1
  s/1 -> Feet Jacobians/1(s)
  w_H_b/1 -> Feet Jacobians/2(w_H_b)
  Feet Jacobians/1(J_LFoot) -> Compute Base Velocity/1(J_LeftFoot)
  Feet Jacobians/2(J_RFoot) -> Compute Base Velocity/2(J_RightFoot)

== system positionWalking_legacy/Dynamics and Kinematics/Inverse Kinematics/ComputeTasksPoseAndVelocity ==
  J_LFoot : Inport
  J_RFoot : Inport  Port=2
  J_CoM : Inport  Port=3
  J_Rot_task : Inport  Port=4
  qj : Inport  Port=5
  w_H_b : Inport  Port=6
  nu : Inport  Port=7
  Compose Task Pose and Velocity : MATLAB Function  TreatAsAtomicUnit=on
      settings: PermitHierarchicalResolution=ParametersOnly
  Product{,1..3} (4 alike) : Product  Multiplication=Matrix(*)
  Task position and orientation : Subsystem
  pos_vel_CoM : Outport
  pose_vel_LFoot : Outport  Port=2
  pose_vel_RFoot : Outport  Port=3
  orient_vel_Rot_task : Outport  Port=4
  wires:
  Compose Task Pose and Velocity/3(pose_vel_RFoot) -> pose_vel_RFoot/1
  Compose Task Pose and Velocity/2(pose_vel_LFoot) -> pose_vel_LFoot/1
  Compose Task Pose and Velocity/1(pos_vel_CoM) -> pos_vel_CoM/1
  Compose Task Pose and Velocity/4(orient_vel_Rot_task) -> orient_vel_Rot_task/1
  nu/1 -> Product1/2, Product/2, Product2/2, Product3/2
  J_Rot_task/1 -> Product3/1
  Product/1 -> Compose Task Pose and Velocity/1(vel_CoM)
  Product1/1 -> Compose Task Pose and Velocity/2(vel_LFoot)
  Product2/1 -> Compose Task Pose and Velocity/3(vel_RFoot)
  Product3/1 -> Compose Task Pose and Velocity/4(vel_Rot_task)
  qj/1 -> Task position and orientation/1(s)
  w_H_b/1 -> Task position and orientation/2(w_H_b)
  Task position and orientation/1(w_H_CoM) -> Compose Task Pose and Velocity/5(w_H_CoM)
  Task position and orientation/2(w_H_l_sole) -> Compose Task Pose and Velocity/6(w_H_l_sole)
  Task position and orientation/3(w_H_r_sole) -> Compose Task Pose and Velocity/7(w_H_r_sole)
  Task position and orientation/4(w_H_Rot_task) -> Compose Task Pose and Velocity/8(w_H_Rot_task)
  J_LFoot/1 -> Product1/1
  J_CoM/1 -> Product/1
  J_RFoot/1 -> Product2/1

== system positionWalking_legacy/Dynamics and Kinematics/Inverse Kinematics/Jacobians and JDot_nu ==
  s : Inport
  w_H_b : Inport  Port=2
  nu_b : Inport  Port=3
  sDot : Inport  Port=4
  DotJ Nu : WBToolboxLibrary/wholeBodyModel/Jacobians/DotJ Nu  frameName=Frames.COM  robotName=WBT_robotName  localName=WBT_modelName  wbiFile=WBT_wbiFilename  wbiList=WBT_wbiList
  DotJ Nu1 : WBToolboxLibrary/wholeBodyModel/Jacobians/DotJ Nu  frameName=Frames.RIGHT_FOOT  robotName=WBT_robotName  localName=WBT_modelName  wbiFile=WBT_wbiFilename  wbiList=WBT_wbiList
  DotJ Nu2 : WBToolboxLibrary/wholeBodyModel/Jacobians/DotJ Nu  frameName=Frames.ROT_TASK_LINK  robotName=WBT_robotName  localName=WBT_modelName  wbiFile=WBT_wbiFilename  wbiList=WBT_wbiList
  DotJ Nu3 : WBToolboxLibrary/wholeBodyModel/Jacobians/DotJ Nu  frameName=Frames.LEFT_FOOT  robotName=WBT_robotName  localName=WBT_modelName  wbiFile=WBT_wbiFilename  wbiList=WBT_wbiList
  Jacobian CoM : WBToolboxLibrary/wholeBodyModel/Jacobians/Jacobian  frameName=Frames.COM  robotName=WBT_robotName  localName=WBT_modelName  wbiFile=WBT_wbiFilename  wbiList=WBT_wbiList
  Jacobian LFoot : WBToolboxLibrary/wholeBodyModel/Jacobians/Jacobian  frameName=Frames.LEFT_FOOT  robotName=WBT_robotName  localName=WBT_modelName  wbiFile=WBT_wbiFilename  wbiList=WBT_wbiList
  Jacobian RFoot : WBToolboxLibrary/wholeBodyModel/Jacobians/Jacobian  frameName=Frames.RIGHT_FOOT  robotName=WBT_robotName  localName=WBT_modelName  wbiFile=WBT_wbiFilename  wbiList=WBT_wbiList
  Jacobian Root Link : WBToolboxLibrary/wholeBodyModel/Jacobians/Jacobian  frameName=Frames.ROT_TASK_LINK  robotName=WBT_robotName  localName=WBT_modelName  wbiFile=WBT_wbiFilename  wbiList=WBT_wbiList
  J_LFoot : Outport
  J_RFoot : Outport  Port=2
  J_CoM : Outport  Port=3
  J_Rot_task : Outport  Port=4
  JDot_nu_LFoot : Outport  Port=5
  JDot_nu_RFoot : Outport  Port=6
  JDot_nu_CoM : Outport  Port=7
  JDot_nu_Rot_task : Outport  Port=8
  wires:
  Jacobian CoM/1 -> J_CoM/1
  Jacobian Root Link/1 -> J_Rot_task/1
  Jacobian LFoot/1 -> J_LFoot/1
  Jacobian RFoot/1 -> J_RFoot/1
  w_H_b/1 -> Jacobian RFoot/1, Jacobian LFoot/1, DotJ Nu1/1, DotJ Nu3/1, DotJ Nu2/1, DotJ Nu/1, Jacobian CoM/1, Jacobian Root Link/1
  sDot/1 -> DotJ Nu1/4, DotJ Nu3/4, DotJ Nu2/4, DotJ Nu/4
  nu_b/1 -> DotJ Nu/3, DotJ Nu1/3, DotJ Nu3/3, DotJ Nu2/3
  s/1 -> DotJ Nu1/2, DotJ Nu3/2, DotJ Nu2/2, DotJ Nu/2, Jacobian RFoot/2, Jacobian CoM/2, Jacobian Root Link/2, Jacobian LFoot/2
  DotJ Nu1/1 -> JDot_nu_RFoot/1
  DotJ Nu3/1 -> JDot_nu_LFoot/1
  DotJ Nu2/1 -> JDot_nu_Rot_task/1
  DotJ Nu/1 -> JDot_nu_CoM/1

== system positionWalking_legacy/Dynamics and Kinematics/Inverse Kinematics/QP-Based Inverse Kinematics ==
  q_0 : Inport
  nu_0 : Inport  Port=2
  s_sDot_sDDot_ref : Inport  Port=3
  J : Inport  Port=4
  JDot_nu : Inport  Port=5
  acc_task_star : Inport  Port=6
  impedances : Inport  Port=7
  dampings : Inport  Port=8
  "Compute QP Hessian, gradient and constraints " : MATLAB Function  TreatAsAtomicUnit=on
      settings: PermitHierarchicalResolution=ParametersOnly
  QP Solver (inverse kinematics) : Subsystem
  Selector3 : Selector  InputPortWidth=ROBOT_DOF+16  IndexOptions=Index vector (dialog)  Indices=[17:ROBOT_DOF+16]  OutputSizes=1
  inverse kinematics integration : Subsystem
  s_sDot_sDDot_des : Outport
  ExitFlagQP : Outport  Port=2
  nuDot : Outport  Port=3
  q : Outport  Port=4
  nu : Outport  Port=5
  wires:
  q_0/1 -> inverse kinematics integration/3(q_0)
  nu_0/1 -> inverse kinematics integration/2(nu_0)
  QP Solver (inverse kinematics)/1(nuDot) -> inverse kinematics integration/1(nuDot), nuDot/1
  "Compute QP Hessian, gradient and constraints "/4(biasVectorConstraint) -> QP Solver (inverse kinematics)/4(biasVectorConstraint)
  "Compute QP Hessian, gradient and constraints "/3(ConstraintMatrix) -> QP Solver (inverse kinematics)/3(ConstraintMatrix)
  "Compute QP Hessian, gradient and constraints "/2(gradient) -> QP Solver (inverse kinematics)/2(gradient)
  "Compute QP Hessian, gradient and constraints "/1(Hessian) -> QP Solver (inverse kinematics)/1(Hessian)
  acc_task_star/1 -> "Compute QP Hessian, gradient and constraints "/8(acc_task_star)
  JDot_nu/1 -> "Compute QP Hessian, gradient and constraints "/7(JDot_nu)
  impedances/1 -> "Compute QP Hessian, gradient and constraints "/4(impedances)
  dampings/1 -> "Compute QP Hessian, gradient and constraints "/5(dampings)
  s_sDot_sDDot_ref/1 -> "Compute QP Hessian, gradient and constraints "/3(s_sDot_sDDot_ref)
  inverse kinematics integration/3(s_sDot_sDDot_des) -> s_sDot_sDDot_des/1
  inverse kinematics integration/2(q) -> q/1, Selector3/1
  Selector3/1 -> "Compute QP Hessian, gradient and constraints "/1(s)
  QP Solver (inverse kinematics)/2(ExitFlagQP) -> ExitFlagQP/1
  J/1 -> "Compute QP Hessian, gradient and constraints "/6(J)
  inverse kinematics integration/1(nu) -> nu/1, "Compute QP Hessian, gradient and constraints "/2(nu)
